simulink model "test_powermode"  (R2015b)
settings: Solver=FixedStepDiscrete  StartTime=0.0  StopTime=Inf  FixedStep=0.001  RelTol=1e-3
PostLoadFcn:
  | , if any(exist('dsrtsu_mdlpostloadfcn', 'file') == [2, 3, 6]), try dsrtsu_mdlpostloadfcn('Execute', bdroot); catch fprintf('Error in PostLoadFcn (dsrtsu_mdlpostloadfcn) for model "%s":\n %s\n', bdroot, lasterr); end, end,
undefined symbols (not defined in the file or in its folder): powermode, PowerMode
settings Model: DSRTSU_INTERNAL_RTI_VER=460  DSRTSU_INTERNAL_RTI_TYPE=rti1401  Creator=luis  LastModifiedBy=luis
settings SolverCC: AutoInsertRateTranBlk=on  InsertRTBMode=Always
settings OptimizationCC: BlockReduction=off  OptimizeBlockIOStorage=off  BufferReuse=off  GlobalBufferReuse=off  ExpressionFolding=off  LocalBlockOutputs=off
settings HardwareCC: ProdEndianess=BigEndian  ProdWordSize=32  ProdHWDeviceType=Generic->Custom  TargetIntDivRoundTo=Zero  TargetEndianess=BigEndian  TargetHWDeviceType=Generic->Custom
settings RTWCC: SystemTargetFile=rti1401.tlc  MakeCommand=make_rti  TemplateMakefile=rti1401.tmf  Description=dSPACE DS1401 Hardware Platform
settings STFCustomTargetCC: ParMdlRefBuildCompliant=on  ConcurrentExecutionCompliant=off  GeneratePreprocessorConditionals=Use local settings  MatFileLogging=on  CPPClassGenCompliant=off  SystemTargetFile=rti1401.tlc
settings GRTTargetCC: CompOptLevelCompliant=off  ConcurrentExecutionCompliant=off  CombineOutputUpdateFcns=off  CPPClassGenCompliant=off  GRTInterface=on  UseToolchainInfoCompliant=off

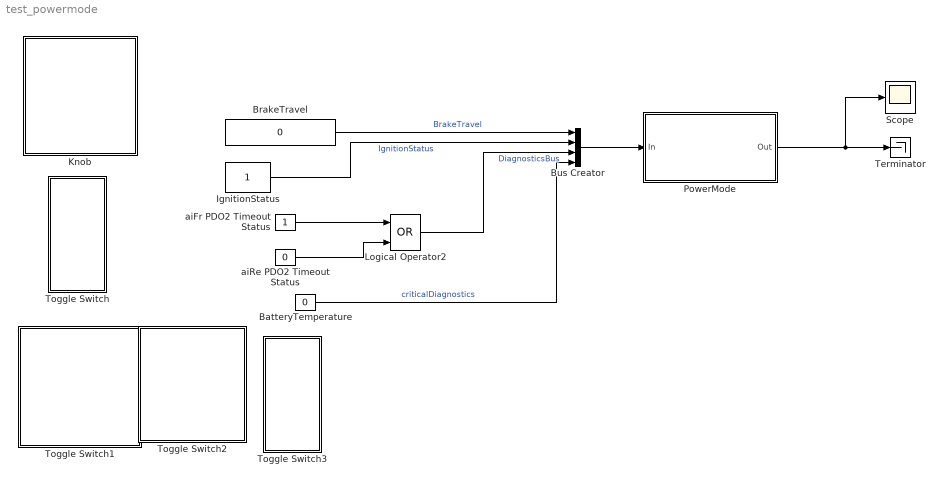
== system test_powermode ==
  BatteryTemperature : Constant  Value=0
  BrakeTravel : Constant  Value=0
  Bus Creator : BusCreator  Inputs=4
  IgnitionStatus : Constant
  Knob : Subsystem  DialogController=hmiCreateDDGDialog  IsWebBlock=on  mask(MWDashboardBlock){webBlockId=d527e6d4-de28-4643-81bd-19861c81b76b, webBlockType=continuousknob, ShowInLibBrowser=on, ShowInitialText=on, HMISrcModelName=test_powermode}
      mask prompts: webBlockId "WebBlock Id"; webBlockType "WebBlock Type"; HMISrcModelName "Source Model"
      mask Help: helpview([docroot '/mapfiles/simulink.map'], 'hmi_knob')
      mask Display:
      | if strcmp(get_param(bdroot(gcb),'BlockDiagramType'), 'library')
      |     image([(matlabroot) '/toolbox/simulink/hmi/icons/ContinuousKnob.png']);
      | end
  Logical Operator2 : Logic  Operator=OR  AllPortsSameDT=off  OutDataTypeStr=boolean
  PowerMode : Subsystem  AncestorBlock=powermode/PowerMode
  Scope : Scope
  Terminator : Terminator
  Toggle Switch : Subsystem  DialogController=hmiCreateDDGDialog  IsWebBlock=on  mask(MWDashboardBlock){webBlockId=24d4186c-734c-4cfd-99e1-c29fb4f67a1f, webBlockType=toggleswitch, ShowInLibBrowser=on, ShowInitialText=on, HMISrcModelName=test_powermode}
      mask prompts: webBlockId "WebBlock Id"; webBlockType "WebBlock Type"; HMISrcModelName "Source Model"
      mask Help: helpview([docroot '/mapfiles/simulink.map'], 'hmi_toggle_switch')
      mask Display:
      | if strcmp(get_param(bdroot(gcb),'BlockDiagramType'), 'library')
      |     image([(matlabroot) '/toolbox/simulink/hmi/icons/ToggleSwitch.png']);
      | end
  Toggle Switch1 : Subsystem  DialogController=hmiCreateDDGDialog  IsWebBlock=on  mask(MWDashboardBlock){webBlockId=8cc6eb90-edda-437e-8ae4-924bab8c4cc0, webBlockType=toggleswitch, ShowInLibBrowser=on, ShowInitialText=on, HMISrcModelName=test_powermode}
      mask prompts: webBlockId "WebBlock Id"; webBlockType "WebBlock Type"; HMISrcModelName "Source Model"
      mask Help: helpview([docroot '/mapfiles/simulink.map'], 'hmi_toggle_switch')
      mask Display:
      | if strcmp(get_param(bdroot(gcb),'BlockDiagramType'), 'library')
      |     image([(matlabroot) '/toolbox/simulink/hmi/icons/ToggleSwitch.png']);
      | end
  Toggle Switch2 : Subsystem  DialogController=hmiCreateDDGDialog  IsWebBlock=on  mask(MWDashboardBlock){webBlockId=ccb7bc30-24cd-4aeb-b352-6e7b8a469afe, webBlockType=toggleswitch, ShowInLibBrowser=on, ShowInitialText=on, HMISrcModelName=test_powermode}
      mask prompts: webBlockId "WebBlock Id"; webBlockType "WebBlock Type"; HMISrcModelName "Source Model"
      mask Help: helpview([docroot '/mapfiles/simulink.map'], 'hmi_toggle_switch')
      mask Display:
      | if strcmp(get_param(bdroot(gcb),'BlockDiagramType'), 'library')
      |     image([(matlabroot) '/toolbox/simulink/hmi/icons/ToggleSwitch.png']);
      | end
  Toggle Switch3 : Subsystem  DialogController=hmiCreateDDGDialog  IsWebBlock=on  mask(MWDashboardBlock){webBlockId=1c47e935-9b96-47b6-920b-1d3775539cc5, webBlockType=toggleswitch, ShowInLibBrowser=on, ShowInitialText=on, HMISrcModelName=test_powermode}
      mask prompts: webBlockId "WebBlock Id"; webBlockType "WebBlock Type"; HMISrcModelName "Source Model"
      mask Help: helpview([docroot '/mapfiles/simulink.map'], 'hmi_toggle_switch')
      mask Display:
      | if strcmp(get_param(bdroot(gcb),'BlockDiagramType'), 'library')
      |     image([(matlabroot) '/toolbox/simulink/hmi/icons/ToggleSwitch.png']);
      | end
  aiFr PDO2 Timeout Status : Constant
  aiRe PDO2 Timeout Status : Constant  Value=0
  wires:
  IgnitionStatus/1 -> Bus Creator/2  "IgnitionStatus"
  Logical Operator2/1 -> Bus Creator/3  "DiagnosticsBus"
  PowerMode/1(Out) -> Scope/1, Terminator/1
  Bus Creator/1 -> PowerMode/1(In)
  BrakeTravel/1 -> Bus Creator/1  "BrakeTravel"
  aiFr PDO2 Timeout Status/1 -> Logical Operator2/1
  aiRe PDO2 Timeout Status/1 -> Logical Operator2/2
  BatteryTemperature/1 -> Bus Creator/4  "criticalDiagnostics"

== system test_powermode/Knob ==

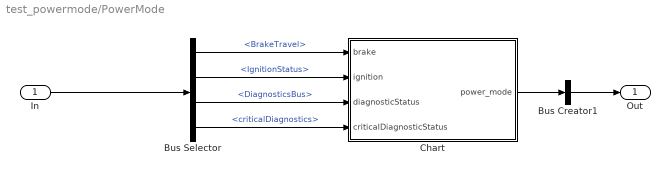
== system test_powermode/PowerMode ==
  In : Inport
  Bus Creator1 : BusCreator  Inputs=1
  Bus Selector : BusSelector  OutputSignals=BrakeTravel,IgnitionStatus,DiagnosticsBus,criticalDiagnostics
  Chart : Stateflow chart  TreatAsAtomicUnit=on
  Out : Outport
  wires:
  Bus Selector/1 -> Chart/1(brake)  "<BrakeTravel>"
  Bus Creator1/1 -> Out/1
  Chart/1(power_mode) -> Bus Creator1/1
  In/1 -> Bus Selector/1
  Bus Selector/3 -> Chart/3(diagnosticStatus)  "<DiagnosticsBus>"
  Bus Selector/2 -> Chart/2(ignition)  "<IgnitionStatus>"
  Bus Selector/4 -> Chart/4(criticalDiagnosticStatus)  "<criticalDiagnostics>"

== system test_powermode/Toggle Switch ==

== system test_powermode/Toggle Switch1 ==

== system test_powermode/Toggle Switch2 ==

== system test_powermode/Toggle Switch3 ==

== stateflow chart test_powermode/PowerMode/Chart ==
  state Startup
    entry:
    power_mode = 0;
    during:
    exit:
  note: Startup
      | Sequence
  state ReadyToDrive
    entry:
    power_mode = 2;
    during:
    exit:
  state PreRTD
  state Idle
    entry:
    power_mode = 1;
    during:
    exit:
  note: Non critical fault
      | Recovered
  state Stopped
    entry:
    power_mode = 4;
    during:
    exit:
  note: Fault
      | Detected
  note: Critical Fault
      | Detected
  state Fault
    entry:
    power_mode = 9;
    during:
    exit:
  (default) -> Startup
  Startup -> Idle : after(2,sec)
  Idle -> PreRTD [order 2] : [brake > 90 && ignition == 0]
  PreRTD -> ReadyToDrive [order 2] : [ignition == 1]
  Fault -> ReadyToDrive [order 2] : [diagnosticStatus ~= 1 ]
  PreRTD -> Idle [order 1] : [brake < 90 || diagnosticStatus == 1 || criticalDiagnosticStatus == 1]
  ReadyToDrive -> Idle [order 2] : [ignition == 0]
  ReadyToDrive -> Fault [order 1] : [diagnosticStatus == 1 || criticalDiagnosticStatus == 1]
  Idle -> Stopped [order 1] : [diagnosticStatus == 1 || criticalDiagnosticStatus == 1]
  Stopped -> Idle : [diagnosticStatus ~= 1 && criticalDiagnosticStatus ~= 1]
  Fault -> Stopped [order 1] : [criticalDiagnosticStatus == 1]
  data: power_mode output double =0; brake input [0..100]; ignition input; diagnosticStatus input; criticalDiagnosticStatus input
